simulink model "gm_parallel_8_prediction_and_cost_function"  (R2022a)
settings: Solver=FixedStepDiscrete  StartTime=0.0  StopTime=10.0  RelTol=1e-3
undefined symbols (not defined in the file or in its folder): f_c, L_d, L_q, L_x, L_y, p, psi_pm, R_ph
libraries: hdlmdlgenlib x42, hdlsllib x5
(part 3 of 7)

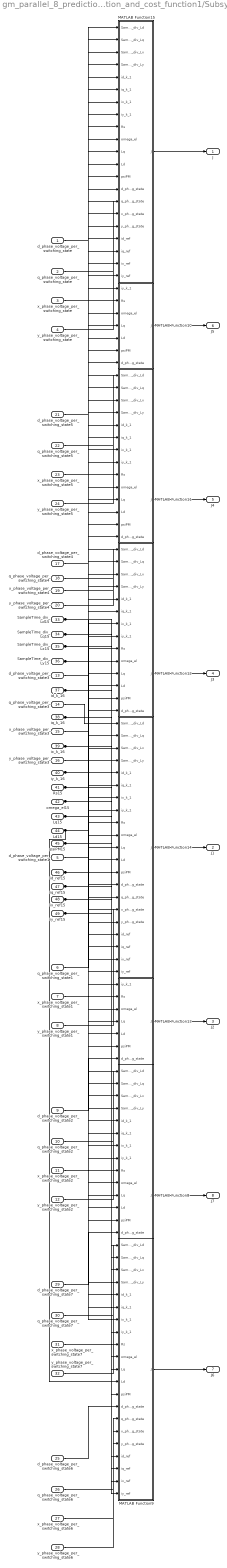
== system gm_parallel_8_prediction_and_cost_function/Prediction_and_cost_function1/Subsystem ==
  d_phase_voltage_per_switching_state : Inport  OutDataTypeStr=single  PortDimensions=1  SampleTime=1e-08
  q_phase_voltage_per_switching_state : Inport  Port=2  OutDataTypeStr=single  PortDimensions=1  SampleTime=1e-08
  x_phase_voltage_per_switching_state : Inport  Port=3  OutDataTypeStr=single  PortDimensions=1  SampleTime=1e-08
  y_phase_voltage_per_switching_state : Inport  Port=4  OutDataTypeStr=single  PortDimensions=1  SampleTime=1e-08
  d_phase_voltage_per_switching_state1 : Inport  Port=5  OutDataTypeStr=single  PortDimensions=1  SampleTime=1e-08
  q_phase_voltage_per_switching_state1 : Inport  Port=6  OutDataTypeStr=single  PortDimensions=1  SampleTime=1e-08
  x_phase_voltage_per_switching_state1 : Inport  Port=7  OutDataTypeStr=single  PortDimensions=1  SampleTime=1e-08
  y_phase_voltage_per_switching_state1 : Inport  Port=8  OutDataTypeStr=single  PortDimensions=1  SampleTime=1e-08
  d_phase_voltage_per_switching_state2 : Inport  Port=9  OutDataTypeStr=single  PortDimensions=1  SampleTime=1e-08
  q_phase_voltage_per_switching_state2 : Inport  Port=10  OutDataTypeStr=single  PortDimensions=1  SampleTime=1e-08
  x_phase_voltage_per_switching_state2 : Inport  Port=11  OutDataTypeStr=single  PortDimensions=1  SampleTime=1e-08
  y_phase_voltage_per_switching_state2 : Inport  Port=12  OutDataTypeStr=single  PortDimensions=1  SampleTime=1e-08
  d_phase_voltage_per_switching_state3 : Inport  Port=13  OutDataTypeStr=single  PortDimensions=1  SampleTime=1e-08
  q_phase_voltage_per_switching_state3 : Inport  Port=14  OutDataTypeStr=single  PortDimensions=1  SampleTime=1e-08
  x_phase_voltage_per_switching_state3 : Inport  Port=15  OutDataTypeStr=single  PortDimensions=1  SampleTime=1e-08
  y_phase_voltage_per_switching_state3 : Inport  Port=16  OutDataTypeStr=single  PortDimensions=1  SampleTime=1e-08
  d_phase_voltage_per_switching_state4 : Inport  Port=17  OutDataTypeStr=single  PortDimensions=1  SampleTime=1e-08
  q_phase_voltage_per_switching_state4 : Inport  Port=18  OutDataTypeStr=single  PortDimensions=1  SampleTime=1e-08
  x_phase_voltage_per_switching_state4 : Inport  Port=19  OutDataTypeStr=single  PortDimensions=1  SampleTime=1e-08
  y_phase_voltage_per_switching_state4 : Inport  Port=20  OutDataTypeStr=single  PortDimensions=1  SampleTime=1e-08
  d_phase_voltage_per_switching_state5 : Inport  Port=21  OutDataTypeStr=single  PortDimensions=1  SampleTime=1e-08
  q_phase_voltage_per_switching_state5 : Inport  Port=22  OutDataTypeStr=single  PortDimensions=1  SampleTime=1e-08
  x_phase_voltage_per_switching_state5 : Inport  Port=23  OutDataTypeStr=single  PortDimensions=1  SampleTime=1e-08
  y_phase_voltage_per_switching_state5 : Inport  Port=24  OutDataTypeStr=single  PortDimensions=1  SampleTime=1e-08
  d_phase_voltage_per_switching_state6 : Inport  Port=25  OutDataTypeStr=single  PortDimensions=1  SampleTime=1e-08
  q_phase_voltage_per_switching_state6 : Inport  Port=26  OutDataTypeStr=single  PortDimensions=1  SampleTime=1e-08
  x_phase_voltage_per_switching_state6 : Inport  Port=27  OutDataTypeStr=single  PortDimensions=1  SampleTime=1e-08
  y_phase_voltage_per_switching_state6 : Inport  Port=28  OutDataTypeStr=single  PortDimensions=1  SampleTime=1e-08
  d_phase_voltage_per_switching_state7 : Inport  Port=29  OutDataTypeStr=single  PortDimensions=1  SampleTime=1e-08
  q_phase_voltage_per_switching_state7 : Inport  Port=30  OutDataTypeStr=single  PortDimensions=1  SampleTime=1e-08
  x_phase_voltage_per_switching_state7 : Inport  Port=31  OutDataTypeStr=single  PortDimensions=1  SampleTime=1e-08
  y_phase_voltage_per_switching_state7 : Inport  Port=32  OutDataTypeStr=single  PortDimensions=1  SampleTime=1e-08
  SampleTime_div_Ld15 : Inport  Port=33  OutDataTypeStr=single  PortDimensions=1  SampleTime=1e-08
  SampleTime_div_Lq15 : Inport  Port=34  OutDataTypeStr=single  PortDimensions=1  SampleTime=1e-08
  SampleTime_div_Lx15 : Inport  Port=35  OutDataTypeStr=single  PortDimensions=1  SampleTime=1e-08
  SampleTime_div_Ly15 : Inport  Port=36  OutDataTypeStr=single  PortDimensions=1  SampleTime=1e-08
  id_k_16 : Inport  Port=37  OutDataTypeStr=single  PortDimensions=1  SampleTime=1e-08
  iq_k_16 : Inport  Port=38  OutDataTypeStr=single  PortDimensions=1  SampleTime=1e-08
  ix_k_16 : Inport  Port=39  OutDataTypeStr=single  PortDimensions=1  SampleTime=1e-08
  iy_k_16 : Inport  Port=40  OutDataTypeStr=single  PortDimensions=1  SampleTime=1e-08
  Rs15 : Inport  Port=41  OutDataTypeStr=single  PortDimensions=1  SampleTime=1e-08
  omega_el15 : Inport  Port=42  OutDataTypeStr=single  PortDimensions=1  SampleTime=1e-08
  Lq15 : Inport  Port=43  OutDataTypeStr=single  PortDimensions=1  SampleTime=1e-08
  Ld15 : Inport  Port=44  OutDataTypeStr=single  PortDimensions=1  SampleTime=1e-08
  psiPM15 : Inport  Port=45  OutDataTypeStr=single  PortDimensions=1  SampleTime=1e-08
  id_ref15 : Inport  Port=46  OutDataTypeStr=single  PortDimensions=1  SampleTime=1e-08
  iq_ref15 : Inport  Port=47  OutDataTypeStr=single  PortDimensions=1  SampleTime=1e-08
  ix_ref15 : Inport  Port=48  OutDataTypeStr=single  PortDimensions=1  SampleTime=1e-08
  iy_ref15 : Inport  Port=49  OutDataTypeStr=single  PortDimensions=1  SampleTime=1e-08
  MATLAB Function10 : Subsystem
  MATLAB Function11 : Subsystem
  MATLAB Function12 : Subsystem
  MATLAB Function13 : Subsystem
  MATLAB Function14 : Subsystem
  MATLAB Function15 : Subsystem
  MATLAB Function8 : Subsystem
  MATLAB Function9 : Subsystem
  J : Outport  SampleTime=1e-08
  J1 : Outport  Port=2  SampleTime=1e-08
  J2 : Outport  Port=3  SampleTime=1e-08
  J3 : Outport  Port=4  SampleTime=1e-08
  J4 : Outport  Port=5  SampleTime=1e-08
  J5 : Outport  Port=6  SampleTime=1e-08
  J6 : Outport  Port=7  SampleTime=1e-08
  J7 : Outport  Port=8  SampleTime=1e-08
  wires:
  MATLAB Function10/1(J) -> J5/1
  MATLAB Function11/1(J) -> J4/1
  MATLAB Function12/1(J) -> J3/1
  MATLAB Function13/1(J) -> J2/1
  MATLAB Function14/1(J) -> J1/1
  MATLAB Function15/1(J) -> J/1
  MATLAB Function8/1(J) -> J7/1
  MATLAB Function9/1(J) -> J6/1
  d_phase_voltage_per_switching_state/1 -> MATLAB Function15/14(d_phase_voltage_per_switching_state)
  q_phase_voltage_per_switching_state/1 -> MATLAB Function15/15(q_phase_voltage_per_switching_state)
  x_phase_voltage_per_switching_state/1 -> MATLAB Function15/16(x_phase_voltage_per_switching_state)
  y_phase_voltage_per_switching_state/1 -> MATLAB Function15/17(y_phase_voltage_per_switching_state)
  d_phase_voltage_per_switching_state1/1 -> MATLAB Function14/14(d_phase_voltage_per_switching_state)
  q_phase_voltage_per_switching_state1/1 -> MATLAB Function14/15(q_phase_voltage_per_switching_state)
  x_phase_voltage_per_switching_state1/1 -> MATLAB Function14/16(x_phase_voltage_per_switching_state)
  y_phase_voltage_per_switching_state1/1 -> MATLAB Function14/17(y_phase_voltage_per_switching_state)
  d_phase_voltage_per_switching_state2/1 -> MATLAB Function13/14(d_phase_voltage_per_switching_state)
  q_phase_voltage_per_switching_state2/1 -> MATLAB Function13/15(q_phase_voltage_per_switching_state)
  x_phase_voltage_per_switching_state2/1 -> MATLAB Function13/16(x_phase_voltage_per_switching_state)
  y_phase_voltage_per_switching_state2/1 -> MATLAB Function13/17(y_phase_voltage_per_switching_state)
  d_phase_voltage_per_switching_state3/1 -> MATLAB Function12/14(d_phase_voltage_per_switching_state)
  q_phase_voltage_per_switching_state3/1 -> MATLAB Function12/15(q_phase_voltage_per_switching_state)
  x_phase_voltage_per_switching_state3/1 -> MATLAB Function12/16(x_phase_voltage_per_switching_state)
  y_phase_voltage_per_switching_state3/1 -> MATLAB Function12/17(y_phase_voltage_per_switching_state)
  d_phase_voltage_per_switching_state4/1 -> MATLAB Function11/14(d_phase_voltage_per_switching_state)
  q_phase_voltage_per_switching_state4/1 -> MATLAB Function11/15(q_phase_voltage_per_switching_state)
  x_phase_voltage_per_switching_state4/1 -> MATLAB Function11/16(x_phase_voltage_per_switching_state)
  y_phase_voltage_per_switching_state4/1 -> MATLAB Function11/17(y_phase_voltage_per_switching_state)
  d_phase_voltage_per_switching_state5/1 -> MATLAB Function10/14(d_phase_voltage_per_switching_state)
  q_phase_voltage_per_switching_state5/1 -> MATLAB Function10/15(q_phase_voltage_per_switching_state)
  x_phase_voltage_per_switching_state5/1 -> MATLAB Function10/16(x_phase_voltage_per_switching_state)
  y_phase_voltage_per_switching_state5/1 -> MATLAB Function10/17(y_phase_voltage_per_switching_state)
  d_phase_voltage_per_switching_state6/1 -> MATLAB Function9/14(d_phase_voltage_per_switching_state)
  q_phase_voltage_per_switching_state6/1 -> MATLAB Function9/15(q_phase_voltage_per_switching_state)
  x_phase_voltage_per_switching_state6/1 -> MATLAB Function9/16(x_phase_voltage_per_switching_state)
  y_phase_voltage_per_switching_state6/1 -> MATLAB Function9/17(y_phase_voltage_per_switching_state)
  d_phase_voltage_per_switching_state7/1 -> MATLAB Function8/14(d_phase_voltage_per_switching_state)
  q_phase_voltage_per_switching_state7/1 -> MATLAB Function8/15(q_phase_voltage_per_switching_state)
  x_phase_voltage_per_switching_state7/1 -> MATLAB Function8/16(x_phase_voltage_per_switching_state)
  y_phase_voltage_per_switching_state7/1 -> MATLAB Function8/17(y_phase_voltage_per_switching_state)
  SampleTime_div_Ld15/1 -> MATLAB Function9/1(SampleTime_div_Ld), MATLAB Function8/1(SampleTime_div_Ld), MATLAB Function15/1(SampleTime_div_Ld), MATLAB Function14/1(SampleTime_div_Ld), MATLAB Function13/1(SampleTime_div_Ld), MATLAB Function12/1(SampleTime_div_Ld), MATLAB Function11/1(SampleTime_div_Ld), MATLAB Function10/1(SampleTime_div_Ld)
  SampleTime_div_Lq15/1 -> MATLAB Function9/2(SampleTime_div_Lq), MATLAB Function8/2(SampleTime_div_Lq), MATLAB Function15/2(SampleTime_div_Lq), MATLAB Function14/2(SampleTime_div_Lq), MATLAB Function13/2(SampleTime_div_Lq), MATLAB Function12/2(SampleTime_div_Lq), MATLAB Function11/2(SampleTime_div_Lq), MATLAB Function10/2(SampleTime_div_Lq)
  SampleTime_div_Lx15/1 -> MATLAB Function9/3(SampleTime_div_Lx), MATLAB Function8/3(SampleTime_div_Lx), MATLAB Function15/3(SampleTime_div_Lx), MATLAB Function14/3(SampleTime_div_Lx), MATLAB Function13/3(SampleTime_div_Lx), MATLAB Function12/3(SampleTime_div_Lx), MATLAB Function11/3(SampleTime_div_Lx), MATLAB Function10/3(SampleTime_div_Lx)
  SampleTime_div_Ly15/1 -> MATLAB Function9/4(SampleTime_div_Ly), MATLAB Function8/4(SampleTime_div_Ly), MATLAB Function15/4(SampleTime_div_Ly), MATLAB Function14/4(SampleTime_div_Ly), MATLAB Function13/4(SampleTime_div_Ly), MATLAB Function12/4(SampleTime_div_Ly), MATLAB Function11/4(SampleTime_div_Ly), MATLAB Function10/4(SampleTime_div_Ly)
  id_k_16/1 -> MATLAB Function9/5(id_k_1), MATLAB Function8/5(id_k_1), MATLAB Function15/5(id_k_1), MATLAB Function14/5(id_k_1), MATLAB Function13/5(id_k_1), MATLAB Function12/5(id_k_1), MATLAB Function11/5(id_k_1), MATLAB Function10/5(id_k_1)
  iq_k_16/1 -> MATLAB Function9/6(iq_k_1), MATLAB Function8/6(iq_k_1), MATLAB Function15/6(iq_k_1), MATLAB Function14/6(iq_k_1), MATLAB Function13/6(iq_k_1), MATLAB Function12/6(iq_k_1), MATLAB Function11/6(iq_k_1), MATLAB Function10/6(iq_k_1)
  ix_k_16/1 -> MATLAB Function9/7(ix_k_1), MATLAB Function8/7(ix_k_1), MATLAB Function15/7(ix_k_1), MATLAB Function14/7(ix_k_1), MATLAB Function13/7(ix_k_1), MATLAB Function12/7(ix_k_1), MATLAB Function11/7(ix_k_1), MATLAB Function10/7(ix_k_1)
  iy_k_16/1 -> MATLAB Function9/8(iy_k_1), MATLAB Function8/8(iy_k_1), MATLAB Function15/8(iy_k_1), MATLAB Function14/8(iy_k_1), MATLAB Function13/8(iy_k_1), MATLAB Function12/8(iy_k_1), MATLAB Function11/8(iy_k_1), MATLAB Function10/8(iy_k_1)
  Rs15/1 -> MATLAB Function9/9(Rs), MATLAB Function8/9(Rs), MATLAB Function15/9(Rs), MATLAB Function14/9(Rs), MATLAB Function13/9(Rs), MATLAB Function12/9(Rs), MATLAB Function11/9(Rs), MATLAB Function10/9(Rs)
  omega_el15/1 -> MATLAB Function9/10(omega_el), MATLAB Function8/10(omega_el), MATLAB Function15/10(omega_el), MATLAB Function14/10(omega_el), MATLAB Function13/10(omega_el), MATLAB Function12/10(omega_el), MATLAB Function11/10(omega_el), MATLAB Function10/10(omega_el)
  Lq15/1 -> MATLAB Function9/11(Lq), MATLAB Function8/11(Lq), MATLAB Function15/11(Lq), MATLAB Function14/11(Lq), MATLAB Function13/11(Lq), MATLAB Function12/11(Lq), MATLAB Function11/11(Lq), MATLAB Function10/11(Lq)
  Ld15/1 -> MATLAB Function9/12(Ld), MATLAB Function8/12(Ld), MATLAB Function15/12(Ld), MATLAB Function14/12(Ld), MATLAB Function13/12(Ld), MATLAB Function12/12(Ld), MATLAB Function11/12(Ld), MATLAB Function10/12(Ld)
  psiPM15/1 -> MATLAB Function9/13(psiPM), MATLAB Function8/13(psiPM), MATLAB Function15/13(psiPM), MATLAB Function14/13(psiPM), MATLAB Function13/13(psiPM), MATLAB Function12/13(psiPM), MATLAB Function11/13(psiPM), MATLAB Function10/13(psiPM)
  id_ref15/1 -> MATLAB Function9/18(id_ref), MATLAB Function8/18(id_ref), MATLAB Function15/18(id_ref), MATLAB Function14/18(id_ref), MATLAB Function13/18(id_ref), MATLAB Function12/18(id_ref), MATLAB Function11/18(id_ref), MATLAB Function10/18(id_ref)
  iq_ref15/1 -> MATLAB Function9/19(iq_ref), MATLAB Function8/19(iq_ref), MATLAB Function15/19(iq_ref), MATLAB Function14/19(iq_ref), MATLAB Function13/19(iq_ref), MATLAB Function12/19(iq_ref), MATLAB Function11/19(iq_ref), MATLAB Function10/19(iq_ref)
  ix_ref15/1 -> MATLAB Function9/20(ix_ref), MATLAB Function8/20(ix_ref), MATLAB Function15/20(ix_ref), MATLAB Function14/20(ix_ref), MATLAB Function13/20(ix_ref), MATLAB Function12/20(ix_ref), MATLAB Function11/20(ix_ref), MATLAB Function10/20(ix_ref)
  iy_ref15/1 -> MATLAB Function9/21(iy_ref), MATLAB Function8/21(iy_ref), MATLAB Function15/21(iy_ref), MATLAB Function14/21(iy_ref), MATLAB Function13/21(iy_ref), MATLAB Function12/21(iy_ref), MATLAB Function11/21(iy_ref), MATLAB Function10/21(iy_ref)

== system gm_parallel_8_prediction_and_cost_function/Prediction_and_cost_function2/Subsystem ==
  d_phase_voltage_per_switching_state : Inport
  q_phase_voltage_per_switching_state : Inport  Port=2
  x_phase_voltage_per_switching_state : Inport  Port=3
  y_phase_voltage_per_switching_state : Inport  Port=4
  d_phase_voltage_per_switching_state1 : Inport  Port=5
  q_phase_voltage_per_switching_state1 : Inport  Port=6
  x_phase_voltage_per_switching_state1 : Inport  Port=7
  y_phase_voltage_per_switching_state1 : Inport  Port=8
  d_phase_voltage_per_switching_state2 : Inport  Port=9
  q_phase_voltage_per_switching_state2 : Inport  Port=10
  x_phase_voltage_per_switching_state2 : Inport  Port=11
  y_phase_voltage_per_switching_state2 : Inport  Port=12
  d_phase_voltage_per_switching_state3 : Inport  Port=13
  q_phase_voltage_per_switching_state3 : Inport  Port=14
  x_phase_voltage_per_switching_state3 : Inport  Port=15
  y_phase_voltage_per_switching_state3 : Inport  Port=16
  d_phase_voltage_per_switching_state4 : Inport  Port=17
  q_phase_voltage_per_switching_state4 : Inport  Port=18
  x_phase_voltage_per_switching_state4 : Inport  Port=19
  y_phase_voltage_per_switching_state4 : Inport  Port=20
  d_phase_voltage_per_switching_state5 : Inport  Port=21
  q_phase_voltage_per_switching_state5 : Inport  Port=22
  x_phase_voltage_per_switching_state5 : Inport  Port=23
  y_phase_voltage_per_switching_state5 : Inport  Port=24
  d_phase_voltage_per_switching_state6 : Inport  Port=25
  q_phase_voltage_per_switching_state6 : Inport  Port=26
  x_phase_voltage_per_switching_state6 : Inport  Port=27
  y_phase_voltage_per_switching_state6 : Inport  Port=28
  d_phase_voltage_per_switching_state7 : Inport  Port=29
  q_phase_voltage_per_switching_state7 : Inport  Port=30
  x_phase_voltage_per_switching_state7 : Inport  Port=31
  y_phase_voltage_per_switching_state7 : Inport  Port=32
  SampleTime_div_Ld15 : Inport  Port=33
  SampleTime_div_Lq15 : Inport  Port=34
  SampleTime_div_Lx15 : Inport  Port=35
  SampleTime_div_Ly15 : Inport  Port=36
  id_k_16 : Inport  Port=37
  iq_k_16 : Inport  Port=38
  ix_k_16 : Inport  Port=39
  iy_k_16 : Inport  Port=40
  Rs15 : Inport  Port=41
  omega_el15 : Inport  Port=42
  Lq15 : Inport  Port=43
  Ld15 : Inport  Port=44
  psiPM15 : Inport  Port=45
  id_ref15 : Inport  Port=46
  iq_ref15 : Inport  Port=47
  ix_ref15 : Inport  Port=48
  iy_ref15 : Inport  Port=49
  MATLAB Function10 : MATLAB Function  TreatAsAtomicUnit=on  SystemSampleTime=1/100000000
  MATLAB Function11 : MATLAB Function  TreatAsAtomicUnit=on  SystemSampleTime=1/100000000
  MATLAB Function12 : MATLAB Function  TreatAsAtomicUnit=on  SystemSampleTime=1/100000000
  MATLAB Function13 : MATLAB Function  TreatAsAtomicUnit=on  SystemSampleTime=1/100000000
  MATLAB Function14 : MATLAB Function  TreatAsAtomicUnit=on  SystemSampleTime=1/100000000
  MATLAB Function15 : MATLAB Function  TreatAsAtomicUnit=on  SystemSampleTime=1/100000000
  MATLAB Function8 : MATLAB Function  TreatAsAtomicUnit=on  SystemSampleTime=1/100000000
  MATLAB Function9 : MATLAB Function  TreatAsAtomicUnit=on  SystemSampleTime=1/100000000
  J : Outport
  J1 : Outport  Port=2
  J2 : Outport  Port=3
  J3 : Outport  Port=4
  J4 : Outport  Port=5
  J5 : Outport  Port=6
  J6 : Outport  Port=7
  J7 : Outport  Port=8
  wires:
  id_k_16/1 -> MATLAB Function15/5(id_k_1), MATLAB Function14/5(id_k_1), MATLAB Function13/5(id_k_1), MATLAB Function12/5(id_k_1), MATLAB Function11/5(id_k_1), MATLAB Function10/5(id_k_1), MATLAB Function9/5(id_k_1), MATLAB Function8/5(id_k_1)
  iq_k_16/1 -> MATLAB Function15/6(iq_k_1), MATLAB Function14/6(iq_k_1), MATLAB Function13/6(iq_k_1), MATLAB Function12/6(iq_k_1), MATLAB Function11/6(iq_k_1), MATLAB Function10/6(iq_k_1), MATLAB Function9/6(iq_k_1), MATLAB Function8/6(iq_k_1)
  ix_k_16/1 -> MATLAB Function15/7(ix_k_1), MATLAB Function14/7(ix_k_1), MATLAB Function13/7(ix_k_1), MATLAB Function12/7(ix_k_1), MATLAB Function11/7(ix_k_1), MATLAB Function10/7(ix_k_1), MATLAB Function9/7(ix_k_1), MATLAB Function8/7(ix_k_1)
  iy_k_16/1 -> MATLAB Function15/8(iy_k_1), MATLAB Function14/8(iy_k_1), MATLAB Function13/8(iy_k_1), MATLAB Function12/8(iy_k_1), MATLAB Function11/8(iy_k_1), MATLAB Function10/8(iy_k_1), MATLAB Function9/8(iy_k_1), MATLAB Function8/8(iy_k_1)
  Ld15/1 -> MATLAB Function15/12(Ld), MATLAB Function14/12(Ld), MATLAB Function13/12(Ld), MATLAB Function12/12(Ld), MATLAB Function11/12(Ld), MATLAB Function10/12(Ld), MATLAB Function9/12(Ld), MATLAB Function8/12(Ld)
  id_ref15/1 -> MATLAB Function15/18(id_ref), MATLAB Function14/18(id_ref), MATLAB Function13/18(id_ref), MATLAB Function12/18(id_ref), MATLAB Function11/18(id_ref), MATLAB Function10/18(id_ref), MATLAB Function9/18(id_ref), MATLAB Function8/18(id_ref)
  iq_ref15/1 -> MATLAB Function15/19(iq_ref), MATLAB Function14/19(iq_ref), MATLAB Function13/19(iq_ref), MATLAB Function12/19(iq_ref), MATLAB Function11/19(iq_ref), MATLAB Function10/19(iq_ref), MATLAB Function9/19(iq_ref), MATLAB Function8/19(iq_ref)
  ix_ref15/1 -> MATLAB Function15/20(ix_ref), MATLAB Function14/20(ix_ref), MATLAB Function13/20(ix_ref), MATLAB Function12/20(ix_ref), MATLAB Function11/20(ix_ref), MATLAB Function10/20(ix_ref), MATLAB Function9/20(ix_ref), MATLAB Function8/20(ix_ref)
  q_phase_voltage_per_switching_state3/1 -> MATLAB Function12/15(q_phase_voltage_per_switching_state)
  y_phase_voltage_per_switching_state3/1 -> MATLAB Function12/17(y_phase_voltage_per_switching_state)
  q_phase_voltage_per_switching_state7/1 -> MATLAB Function8/15(q_phase_voltage_per_switching_state)
  MATLAB Function12/1(J) -> J3/1
  MATLAB Function9/1(J) -> J6/1
  x_phase_voltage_per_switching_state6/1 -> MATLAB Function9/16(x_phase_voltage_per_switching_state)
  y_phase_voltage_per_switching_state6/1 -> MATLAB Function9/17(y_phase_voltage_per_switching_state)
  q_phase_voltage_per_switching_state6/1 -> MATLAB Function9/15(q_phase_voltage_per_switching_state)
  y_phase_voltage_per_switching_state5/1 -> MATLAB Function10/17(y_phase_voltage_per_switching_state)
  MATLAB Function10/1(J) -> J5/1
  d_phase_voltage_per_switching_state5/1 -> MATLAB Function10/14(d_phase_voltage_per_switching_state)
  MATLAB Function15/1(J) -> J/1
  q_phase_voltage_per_switching_state/1 -> MATLAB Function15/15(q_phase_voltage_per_switching_state)
  x_phase_voltage_per_switching_state7/1 -> MATLAB Function8/16(x_phase_voltage_per_switching_state)
  SampleTime_div_Lq15/1 -> MATLAB Function15/2(SampleTime_div_Lq), MATLAB Function14/2(SampleTime_div_Lq), MATLAB Function13/2(SampleTime_div_Lq), MATLAB Function12/2(SampleTime_div_Lq), MATLAB Function11/2(SampleTime_div_Lq), MATLAB Function10/2(SampleTime_div_Lq), MATLAB Function9/2(SampleTime_div_Lq), MATLAB Function8/2(SampleTime_div_Lq)
  SampleTime_div_Ly15/1 -> MATLAB Function15/4(SampleTime_div_Ly), MATLAB Function14/4(SampleTime_div_Ly), MATLAB Function13/4(SampleTime_div_Ly), MATLAB Function12/4(SampleTime_div_Ly), MATLAB Function11/4(SampleTime_div_Ly), MATLAB Function10/4(SampleTime_div_Ly), MATLAB Function9/4(SampleTime_div_Ly), MATLAB Function8/4(SampleTime_div_Ly)
  SampleTime_div_Lx15/1 -> MATLAB Function15/3(SampleTime_div_Lx), MATLAB Function14/3(SampleTime_div_Lx), MATLAB Function13/3(SampleTime_div_Lx), MATLAB Function12/3(SampleTime_div_Lx), MATLAB Function11/3(SampleTime_div_Lx), MATLAB Function10/3(SampleTime_div_Lx), MATLAB Function9/3(SampleTime_div_Lx), MATLAB Function8/3(SampleTime_div_Lx)
  x_phase_voltage_per_switching_state5/1 -> MATLAB Function10/16(x_phase_voltage_per_switching_state)
  q_phase_voltage_per_switching_state4/1 -> MATLAB Function11/15(q_phase_voltage_per_switching_state)
  d_phase_voltage_per_switching_state4/1 -> MATLAB Function11/14(d_phase_voltage_per_switching_state)
  d_phase_voltage_per_switching_state7/1 -> MATLAB Function8/14(d_phase_voltage_per_switching_state)
  q_phase_voltage_per_switching_state5/1 -> MATLAB Function10/15(q_phase_voltage_per_switching_state)
  x_phase_voltage_per_switching_state/1 -> MATLAB Function15/16(x_phase_voltage_per_switching_state)
  y_phase_voltage_per_switching_state4/1 -> MATLAB Function11/17(y_phase_voltage_per_switching_state)
  MATLAB Function13/1(J) -> J2/1
  x_phase_voltage_per_switching_state2/1 -> MATLAB Function13/16(x_phase_voltage_per_switching_state)
  q_phase_voltage_per_switching_state2/1 -> MATLAB Function13/15(q_phase_voltage_per_switching_state)
  MATLAB Function8/1(J) -> J7/1
  MATLAB Function14/1(J) -> J1/1
  y_phase_voltage_per_switching_state1/1 -> MATLAB Function14/17(y_phase_voltage_per_switching_state)
  x_phase_voltage_per_switching_state4/1 -> MATLAB Function11/16(x_phase_voltage_per_switching_state)
  d_phase_voltage_per_switching_state2/1 -> MATLAB Function13/14(d_phase_voltage_per_switching_state)
  x_phase_voltage_per_switching_state3/1 -> MATLAB Function12/16(x_phase_voltage_per_switching_state)
  d_phase_voltage_per_switching_state/1 -> MATLAB Function15/14(d_phase_voltage_per_switching_state)
  d_phase_voltage_per_switching_state6/1 -> MATLAB Function9/14(d_phase_voltage_per_switching_state)
  d_phase_voltage_per_switching_state3/1 -> MATLAB Function12/14(d_phase_voltage_per_switching_state)
  psiPM15/1 -> MATLAB Function15/13(psiPM), MATLAB Function14/13(psiPM), MATLAB Function13/13(psiPM), MATLAB Function12/13(psiPM), MATLAB Function11/13(psiPM), MATLAB Function10/13(psiPM), MATLAB Function9/13(psiPM), MATLAB Function8/13(psiPM)
  omega_el15/1 -> MATLAB Function15/10(omega_el), MATLAB Function14/10(omega_el), MATLAB Function13/10(omega_el), MATLAB Function12/10(omega_el), MATLAB Function11/10(omega_el), MATLAB Function10/10(omega_el), MATLAB Function9/10(omega_el), MATLAB Function8/10(omega_el)
  iy_ref15/1 -> MATLAB Function15/21(iy_ref), MATLAB Function14/21(iy_ref), MATLAB Function13/21(iy_ref), MATLAB Function12/21(iy_ref), MATLAB Function11/21(iy_ref), MATLAB Function10/21(iy_ref), MATLAB Function9/21(iy_ref), MATLAB Function8/21(iy_ref)
  y_phase_voltage_per_switching_state7/1 -> MATLAB Function8/17(y_phase_voltage_per_switching_state)
  x_phase_voltage_per_switching_state1/1 -> MATLAB Function14/16(x_phase_voltage_per_switching_state)
  d_phase_voltage_per_switching_state1/1 -> MATLAB Function14/14(d_phase_voltage_per_switching_state)
  y_phase_voltage_per_switching_state2/1 -> MATLAB Function13/17(y_phase_voltage_per_switching_state)
  MATLAB Function11/1(J) -> J4/1
  Lq15/1 -> MATLAB Function15/11(Lq), MATLAB Function14/11(Lq), MATLAB Function13/11(Lq), MATLAB Function12/11(Lq), MATLAB Function11/11(Lq), MATLAB Function10/11(Lq), MATLAB Function9/11(Lq), MATLAB Function8/11(Lq)
  y_phase_voltage_per_switching_state/1 -> MATLAB Function15/17(y_phase_voltage_per_switching_state)
  Rs15/1 -> MATLAB Function15/9(Rs), MATLAB Function14/9(Rs), MATLAB Function13/9(Rs), MATLAB Function12/9(Rs), MATLAB Function11/9(Rs), MATLAB Function10/9(Rs), MATLAB Function9/9(Rs), MATLAB Function8/9(Rs)
  SampleTime_div_Ld15/1 -> MATLAB Function15/1(SampleTime_div_Ld), MATLAB Function14/1(SampleTime_div_Ld), MATLAB Function13/1(SampleTime_div_Ld), MATLAB Function12/1(SampleTime_div_Ld), MATLAB Function11/1(SampleTime_div_Ld), MATLAB Function10/1(SampleTime_div_Ld), MATLAB Function9/1(SampleTime_div_Ld), MATLAB Function8/1(SampleTime_div_Ld)
  q_phase_voltage_per_switching_state1/1 -> MATLAB Function14/15(q_phase_voltage_per_switching_state)

== system gm_parallel_8_prediction_and_cost_function/Prediction_and_cost_function1/Detect Rise Positive/Positive ==
  u : Inport  OutDataTypeStr=boolean  SampleTime=1e-08
  Compare : RelationalOperator  Operator=>  OutDataTypeStr=boolean  ZeroCross=off
  Constant : Constant  DisableCoverage=on  Value=0  OutDataTypeStr=Inherit: Inherit via back propagation  SampleTime=-1  PreserveConstantTs=on
  y : Outport  SampleTime=1e-08
  wires:
  Compare/1 -> y/1
  Constant/1 -> Compare/2
  u/1 -> Compare/1

== system gm_parallel_8_prediction_and_cost_function/Prediction_and_cost_function1/Detect Rise Positive1/Positive ==
  u : Inport  OutDataTypeStr=boolean  SampleTime=1e-08
  Compare : RelationalOperator  Operator=>  OutDataTypeStr=boolean  ZeroCross=off
  Constant : Constant  DisableCoverage=on  Value=0  OutDataTypeStr=Inherit: Inherit via back propagation  SampleTime=-1  PreserveConstantTs=on
  y : Outport  SampleTime=1e-08
  wires:
  Compare/1 -> y/1
  Constant/1 -> Compare/2
  u/1 -> Compare/1

== system gm_parallel_8_prediction_and_cost_function/Prediction_and_cost_function1/Detect Rise Positive2/Positive ==
  u : Inport  OutDataTypeStr=boolean  SampleTime=1e-08
  Compare : RelationalOperator  Operator=>  OutDataTypeStr=boolean  ZeroCross=off
  Constant : Constant  DisableCoverage=on  Value=0  OutDataTypeStr=Inherit: Inherit via back propagation  SampleTime=-1  PreserveConstantTs=on
  y : Outport  SampleTime=1e-08
  wires:
  Compare/1 -> y/1
  Constant/1 -> Compare/2
  u/1 -> Compare/1

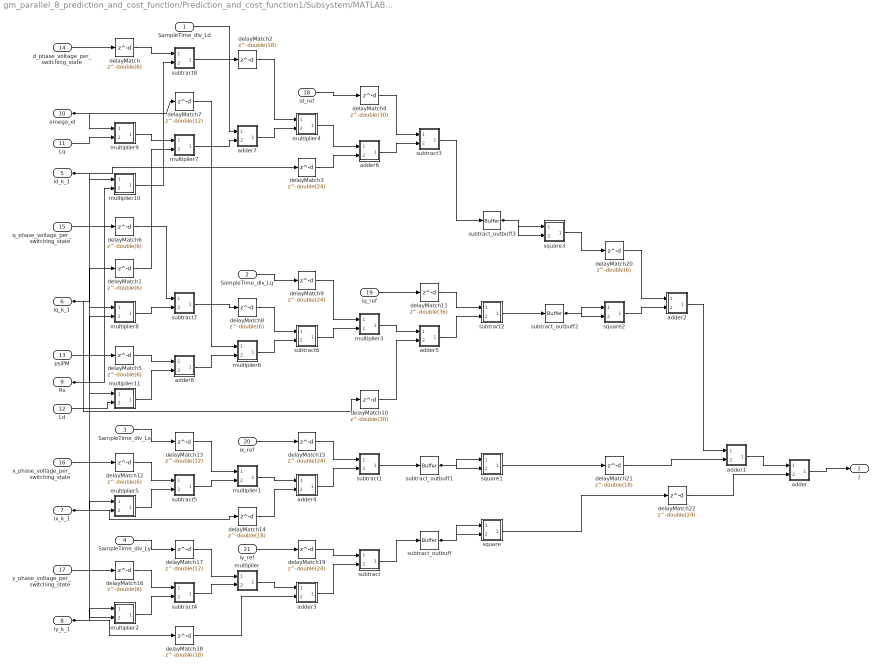
== system gm_parallel_8_prediction_and_cost_function/Prediction_and_cost_function1/Subsystem/MATLAB Function10 ==
  SampleTime_div_Ld : Inport  OutDataTypeStr=single  PortDimensions=1  SampleTime=1e-08
  SampleTime_div_Lq : Inport  Port=2  OutDataTypeStr=single  PortDimensions=1  SampleTime=1e-08
  SampleTime_div_Lx : Inport  Port=3  OutDataTypeStr=single  PortDimensions=1  SampleTime=1e-08
  SampleTime_div_Ly : Inport  Port=4  OutDataTypeStr=single  PortDimensions=1  SampleTime=1e-08
  id_k_1 : Inport  Port=5  OutDataTypeStr=single  PortDimensions=1  SampleTime=1e-08
  iq_k_1 : Inport  Port=6  OutDataTypeStr=single  PortDimensions=1  SampleTime=1e-08
  ix_k_1 : Inport  Port=7  OutDataTypeStr=single  PortDimensions=1  SampleTime=1e-08
  iy_k_1 : Inport  Port=8  OutDataTypeStr=single  PortDimensions=1  SampleTime=1e-08
  Rs : Inport  Port=9  OutDataTypeStr=single  PortDimensions=1  SampleTime=1e-08
  omega_el : Inport  Port=10  OutDataTypeStr=single  PortDimensions=1  SampleTime=1e-08
  Lq : Inport  Port=11  OutDataTypeStr=single  PortDimensions=1  SampleTime=1e-08
  Ld : Inport  Port=12  OutDataTypeStr=single  PortDimensions=1  SampleTime=1e-08
  psiPM : Inport  Port=13  OutDataTypeStr=single  PortDimensions=1  SampleTime=1e-08
  d_phase_voltage_per_switching_state : Inport  Port=14  OutDataTypeStr=single  PortDimensions=1  SampleTime=1e-08
  q_phase_voltage_per_switching_state : Inport  Port=15  OutDataTypeStr=single  PortDimensions=1  SampleTime=1e-08
  x_phase_voltage_per_switching_state : Inport  Port=16  OutDataTypeStr=single  PortDimensions=1  SampleTime=1e-08
  y_phase_voltage_per_switching_state : Inport  Port=17  OutDataTypeStr=single  PortDimensions=1  SampleTime=1e-08
  id_ref : Inport  Port=18  OutDataTypeStr=single  PortDimensions=1  SampleTime=1e-08
  iq_ref : Inport  Port=19  OutDataTypeStr=single  PortDimensions=1  SampleTime=1e-08
  ix_ref : Inport  Port=20  OutDataTypeStr=single  PortDimensions=1  SampleTime=1e-08
  iy_ref : Inport  Port=21  OutDataTypeStr=single  PortDimensions=1  SampleTime=1e-08
  adder : Subsystem
      mask Display: disp('NFP\nadd');
  adder1 : Subsystem
      mask Display: disp('NFP\nadd');
  adder2 : Subsystem
      mask Display: disp('NFP\nadd');
  adder3 : Subsystem
      mask Display: disp('NFP\nadd');
  adder4 : Subsystem
      mask Display: disp('NFP\nadd');
  adder5 : Subsystem
      mask Display: disp('NFP\nadd');
  adder6 : Subsystem
      mask Display: disp('NFP\nadd');
  adder7 : Subsystem
      mask Display: disp('NFP\nadd');
  adder8 : Subsystem
      mask Display: disp('NFP\nadd');
  delayMatch{,1,5..6,8,12,16,20} (8 alike) : Delay  DelayLength=double(6)  InitialCondition=0  SampleTime=1e-08
  delayMatch10 : Delay  DelayLength=double(30)  InitialCondition=0  SampleTime=1e-08
  delayMatch11 : Delay  DelayLength=double(36)  InitialCondition=0  SampleTime=1e-08
  delayMatch13 : Delay  DelayLength=double(12)  InitialCondition=0  SampleTime=1e-08
  delayMatch{2,14,18,21} (4 alike) : Delay  DelayLength=double(18)  InitialCondition=0  SampleTime=1e-08
  delayMatch{3,9,15,19,22} (5 alike) : Delay  DelayLength=double(24)  InitialCondition=0  SampleTime=1e-08
  delayMatch17 : Delay  DelayLength=double(12)  InitialCondition=0  SampleTime=1e-08
  delayMatch4 : Delay  DelayLength=double(30)  InitialCondition=0  SampleTime=1e-08
  delayMatch7 : Delay  DelayLength=double(12)  InitialCondition=0  SampleTime=1e-08
  multiplier : Subsystem
      mask Display: disp('NFP\nmul');
  multiplier1 : Subsystem
      mask Display: disp('NFP\nmul');
  multiplier10 : Subsystem
      mask Display: disp('NFP\nmul');
  multiplier11 : Subsystem
      mask Display: disp('NFP\nmul');
  multiplier2 : Subsystem
      mask Display: disp('NFP\nmul');
  multiplier3 : Subsystem
      mask Display: disp('NFP\nmul');
  multiplier4 : Subsystem
      mask Display: disp('NFP\nmul');
  multiplier5 : Subsystem
      mask Display: disp('NFP\nmul');
  multiplier6 : Subsystem
      mask Display: disp('NFP\nmul');
  multiplier7 : Subsystem
      mask Display: disp('NFP\nmul');
  multiplier8 : Subsystem
      mask Display: disp('NFP\nmul');
  multiplier9 : Subsystem
      mask Display: disp('NFP\nmul');
  square : Subsystem
      mask Display: disp('NFP\nmul');
  square1 : Subsystem
      mask Display: disp('NFP\nmul');
  square2 : Subsystem
      mask Display: disp('NFP\nmul');
  square3 : Subsystem
      mask Display: disp('NFP\nmul');
  subtract : Subsystem
      mask Display: disp('NFP\nadd');
  subtract1 : Subsystem
      mask Display: disp('NFP\nadd');
  subtract2 : Subsystem
      mask Display: disp('NFP\nadd');
  subtract3 : Subsystem
      mask Display: disp('NFP\nadd');
  subtract4 : Subsystem
      mask Display: disp('NFP\nadd');
  subtract5 : Subsystem
      mask Display: disp('NFP\nadd');
  subtract6 : Subsystem
      mask Display: disp('NFP\nadd');
  subtract7 : Subsystem
      mask Display: disp('NFP\nadd');
  subtract8 : Subsystem
      mask Display: disp('NFP\nadd');
  subtract_outbuff{,1..3} (4 alike) : hdlmdlgenlib/Buffer
      settings: SourceProductBaseCode=SL
  J : Outport  SampleTime=1e-08  VectorParamsAs1DForOutWhenUnconnected=off
  wires:
  delayMatch2/1 -> multiplier4/1(In1)
  delayMatch9/1 -> multiplier3/1(In1)
  delayMatch13/1 -> multiplier1/1(In1)
  delayMatch17/1 -> multiplier/1(In1)
  delayMatch3/1 -> adder6/2(In2)
  delayMatch1/1 -> multiplier7/2(In2)
  delayMatch14/1 -> adder4/2(In2)
  delayMatch18/1 -> adder3/2(In2)
  delayMatch7/1 -> multiplier6/1(In1)
  delayMatch5/1 -> adder8/1(In1)
  delayMatch/1 -> subtract8/1(In1)
  delayMatch6/1 -> subtract7/1(In1)
  delayMatch12/1 -> subtract5/1(In1)
  delayMatch16/1 -> subtract4/1(In1)
  delayMatch4/1 -> subtract3/1(In1)
  delayMatch11/1 -> subtract2/1(In1)
  delayMatch15/1 -> subtract1/1(In1)
  delayMatch19/1 -> subtract/1(In1)
  delayMatch22/1 -> adder/2(In2)
  subtract_outbuff/1 -> square/2(In2), square/1(In1)
  delayMatch21/1 -> adder1/2(In2)
  subtract_outbuff1/1 -> square1/2(In2), square1/1(In1)
  delayMatch20/1 -> adder2/1(In1)
  subtract_outbuff2/1 -> square2/2(In2), square2/1(In1)
  subtract_outbuff3/1 -> square3/2(In2), square3/1(In1)
  delayMatch8/1 -> subtract6/1(In1)
  adder/1(Out1) -> J/1
  square/1(Out1) -> delayMatch22/1
  adder1/1(Out1) -> adder/1(In1)
  subtract/1(Out1) -> subtract_outbuff/1
  square1/1(Out1) -> delayMatch21/1
  adder2/1(Out1) -> adder1/1(In1)
  adder3/1(Out1) -> subtract/2(In2)
  subtract1/1(Out1) -> subtract_outbuff1/1
  square2/1(Out1) -> adder2/2(In2)
  square3/1(Out1) -> delayMatch20/1
  multiplier/1(Out1) -> adder3/1(In1)
  adder4/1(Out1) -> subtract1/2(In2)
  subtract2/1(Out1) -> subtract_outbuff2/1
  subtract3/1(Out1) -> subtract_outbuff3/1
  subtract4/1(Out1) -> multiplier/2(In2)
  multiplier1/1(Out1) -> adder4/1(In1)
  adder5/1(Out1) -> subtract2/2(In2)
  adder6/1(Out1) -> subtract3/2(In2)
  multiplier2/1(Out1) -> subtract4/2(In2)
  subtract5/1(Out1) -> multiplier1/2(In2)
  multiplier3/1(Out1) -> adder5/1(In1)
  multiplier4/1(Out1) -> adder6/1(In1)
  multiplier5/1(Out1) -> subtract5/2(In2)
  subtract6/1(Out1) -> multiplier3/2(In2)
  adder7/1(Out1) -> multiplier4/2(In2)
  multiplier6/1(Out1) -> subtract6/2(In2)
  subtract7/1(Out1) -> delayMatch8/1
  multiplier7/1(Out1) -> adder7/2(In2)
  subtract8/1(Out1) -> adder7/1(In1)
  adder8/1(Out1) -> multiplier6/2(In2)
  multiplier8/1(Out1) -> subtract7/2(In2)
  multiplier9/1(Out1) -> multiplier7/1(In1)
  multiplier10/1(Out1) -> subtract8/2(In2)
  multiplier11/1(Out1) -> adder8/2(In2)
  delayMatch10/1 -> adder5/2(In2)
  SampleTime_div_Ld/1 -> delayMatch2/1
  SampleTime_div_Lq/1 -> delayMatch9/1
  SampleTime_div_Lx/1 -> delayMatch13/1
  SampleTime_div_Ly/1 -> delayMatch17/1
  id_k_1/1 -> delayMatch3/1, multiplier11/1(In1), multiplier10/1(In1)
  iq_k_1/1 -> delayMatch10/1, delayMatch1/1, multiplier8/1(In1)
  ix_k_1/1 -> delayMatch14/1, multiplier5/1(In1)
  iy_k_1/1 -> delayMatch18/1, multiplier2/1(In1)
  Rs/1 -> multiplier10/2(In2), multiplier8/2(In2), multiplier5/2(In2), multiplier2/2(In2)
  omega_el/1 -> delayMatch7/1, multiplier9/1(In1)
  Lq/1 -> multiplier9/2(In2)
  Ld/1 -> multiplier11/2(In2)
  psiPM/1 -> delayMatch5/1
  d_phase_voltage_per_switching_state/1 -> delayMatch/1
  q_phase_voltage_per_switching_state/1 -> delayMatch6/1
  x_phase_voltage_per_switching_state/1 -> delayMatch12/1
  y_phase_voltage_per_switching_state/1 -> delayMatch16/1
  id_ref/1 -> delayMatch4/1
  iq_ref/1 -> delayMatch11/1
  ix_ref/1 -> delayMatch15/1
  iy_ref/1 -> delayMatch19/1

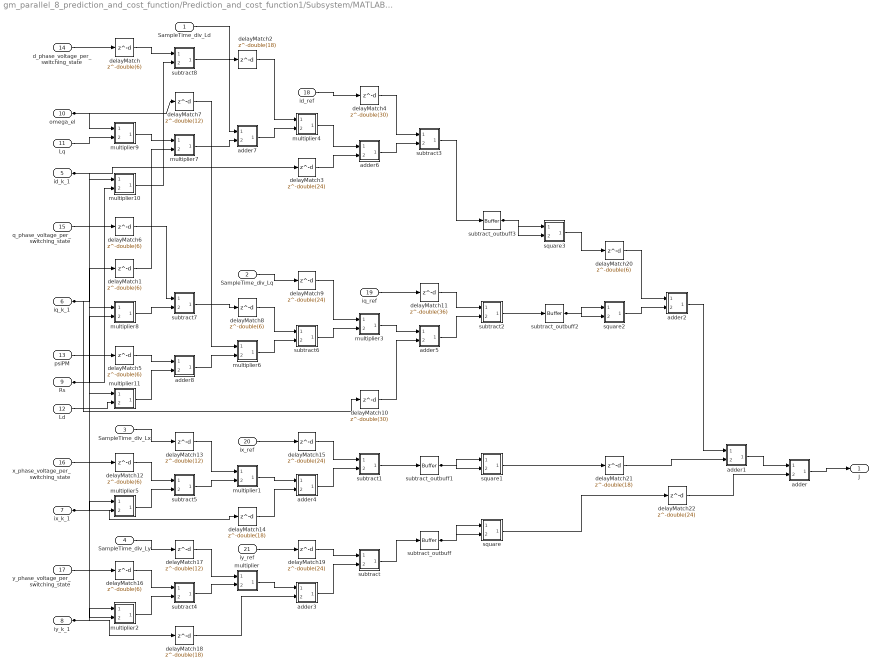
== system gm_parallel_8_prediction_and_cost_function/Prediction_and_cost_function1/Subsystem/MATLAB Function11 ==
  SampleTime_div_Ld : Inport  OutDataTypeStr=single  PortDimensions=1  SampleTime=1e-08
  SampleTime_div_Lq : Inport  Port=2  OutDataTypeStr=single  PortDimensions=1  SampleTime=1e-08
  SampleTime_div_Lx : Inport  Port=3  OutDataTypeStr=single  PortDimensions=1  SampleTime=1e-08
  SampleTime_div_Ly : Inport  Port=4  OutDataTypeStr=single  PortDimensions=1  SampleTime=1e-08
  id_k_1 : Inport  Port=5  OutDataTypeStr=single  PortDimensions=1  SampleTime=1e-08
  iq_k_1 : Inport  Port=6  OutDataTypeStr=single  PortDimensions=1  SampleTime=1e-08
  ix_k_1 : Inport  Port=7  OutDataTypeStr=single  PortDimensions=1  SampleTime=1e-08
  iy_k_1 : Inport  Port=8  OutDataTypeStr=single  PortDimensions=1  SampleTime=1e-08
  Rs : Inport  Port=9  OutDataTypeStr=single  PortDimensions=1  SampleTime=1e-08
  omega_el : Inport  Port=10  OutDataTypeStr=single  PortDimensions=1  SampleTime=1e-08
  Lq : Inport  Port=11  OutDataTypeStr=single  PortDimensions=1  SampleTime=1e-08
  Ld : Inport  Port=12  OutDataTypeStr=single  PortDimensions=1  SampleTime=1e-08
  psiPM : Inport  Port=13  OutDataTypeStr=single  PortDimensions=1  SampleTime=1e-08
  d_phase_voltage_per_switching_state : Inport  Port=14  OutDataTypeStr=single  PortDimensions=1  SampleTime=1e-08
  q_phase_voltage_per_switching_state : Inport  Port=15  OutDataTypeStr=single  PortDimensions=1  SampleTime=1e-08
  x_phase_voltage_per_switching_state : Inport  Port=16  OutDataTypeStr=single  PortDimensions=1  SampleTime=1e-08
  y_phase_voltage_per_switching_state : Inport  Port=17  OutDataTypeStr=single  PortDimensions=1  SampleTime=1e-08
  id_ref : Inport  Port=18  OutDataTypeStr=single  PortDimensions=1  SampleTime=1e-08
  iq_ref : Inport  Port=19  OutDataTypeStr=single  PortDimensions=1  SampleTime=1e-08
  ix_ref : Inport  Port=20  OutDataTypeStr=single  PortDimensions=1  SampleTime=1e-08
  iy_ref : Inport  Port=21  OutDataTypeStr=single  PortDimensions=1  SampleTime=1e-08
  adder : Subsystem
      mask Display: disp('NFP\nadd');
  adder1 : Subsystem
      mask Display: disp('NFP\nadd');
  adder2 : Subsystem
      mask Display: disp('NFP\nadd');
  adder3 : Subsystem
      mask Display: disp('NFP\nadd');
  adder4 : Subsystem
      mask Display: disp('NFP\nadd');
  adder5 : Subsystem
      mask Display: disp('NFP\nadd');
  adder6 : Subsystem
      mask Display: disp('NFP\nadd');
  adder7 : Subsystem
      mask Display: disp('NFP\nadd');
  adder8 : Subsystem
      mask Display: disp('NFP\nadd');
  delayMatch{,1,5..6,8,12,16,20} (8 alike) : Delay  DelayLength=double(6)  InitialCondition=0  SampleTime=1e-08
  delayMatch10 : Delay  DelayLength=double(30)  InitialCondition=0  SampleTime=1e-08
  delayMatch11 : Delay  DelayLength=double(36)  InitialCondition=0  SampleTime=1e-08
  delayMatch13 : Delay  DelayLength=double(12)  InitialCondition=0  SampleTime=1e-08
  delayMatch{2,14,18,21} (4 alike) : Delay  DelayLength=double(18)  InitialCondition=0  SampleTime=1e-08
  delayMatch{3,9,15,19,22} (5 alike) : Delay  DelayLength=double(24)  InitialCondition=0  SampleTime=1e-08
  delayMatch17 : Delay  DelayLength=double(12)  InitialCondition=0  SampleTime=1e-08
  delayMatch4 : Delay  DelayLength=double(30)  InitialCondition=0  SampleTime=1e-08
  delayMatch7 : Delay  DelayLength=double(12)  InitialCondition=0  SampleTime=1e-08
  multiplier : Subsystem
      mask Display: disp('NFP\nmul');
  multiplier1 : Subsystem
      mask Display: disp('NFP\nmul');
  multiplier10 : Subsystem
      mask Display: disp('NFP\nmul');
  multiplier11 : Subsystem
      mask Display: disp('NFP\nmul');
  multiplier2 : Subsystem
      mask Display: disp('NFP\nmul');
  multiplier3 : Subsystem
      mask Display: disp('NFP\nmul');
  multiplier4 : Subsystem
      mask Display: disp('NFP\nmul');
  multiplier5 : Subsystem
      mask Display: disp('NFP\nmul');
  multiplier6 : Subsystem
      mask Display: disp('NFP\nmul');
  multiplier7 : Subsystem
      mask Display: disp('NFP\nmul');
  multiplier8 : Subsystem
      mask Display: disp('NFP\nmul');
  multiplier9 : Subsystem
      mask Display: disp('NFP\nmul');
  square : Subsystem
      mask Display: disp('NFP\nmul');
  square1 : Subsystem
      mask Display: disp('NFP\nmul');
  square2 : Subsystem
      mask Display: disp('NFP\nmul');
  square3 : Subsystem
      mask Display: disp('NFP\nmul');
  subtract : Subsystem
      mask Display: disp('NFP\nadd');
  subtract1 : Subsystem
      mask Display: disp('NFP\nadd');
  subtract2 : Subsystem
      mask Display: disp('NFP\nadd');
  subtract3 : Subsystem
      mask Display: disp('NFP\nadd');
  subtract4 : Subsystem
      mask Display: disp('NFP\nadd');
  subtract5 : Subsystem
      mask Display: disp('NFP\nadd');
  subtract6 : Subsystem
      mask Display: disp('NFP\nadd');
  subtract7 : Subsystem
      mask Display: disp('NFP\nadd');
  subtract8 : Subsystem
      mask Display: disp('NFP\nadd');
  subtract_outbuff{,1..3} (4 alike) : hdlmdlgenlib/Buffer
      settings: SourceProductBaseCode=SL
  J : Outport  SampleTime=1e-08  VectorParamsAs1DForOutWhenUnconnected=off
  wires:
  iy_ref/1 -> delayMatch19/1
  ix_ref/1 -> delayMatch15/1
  iq_ref/1 -> delayMatch11/1
  id_ref/1 -> delayMatch4/1
  y_phase_voltage_per_switching_state/1 -> delayMatch16/1
  x_phase_voltage_per_switching_state/1 -> delayMatch12/1
  q_phase_voltage_per_switching_state/1 -> delayMatch6/1
  d_phase_voltage_per_switching_state/1 -> delayMatch/1
  psiPM/1 -> delayMatch5/1
  Ld/1 -> multiplier11/2(In2)
  Lq/1 -> multiplier9/2(In2)
  omega_el/1 -> multiplier9/1(In1), delayMatch7/1
  Rs/1 -> multiplier2/2(In2), multiplier5/2(In2), multiplier8/2(In2), multiplier10/2(In2)
  iy_k_1/1 -> multiplier2/1(In1), delayMatch18/1
  ix_k_1/1 -> multiplier5/1(In1), delayMatch14/1
  iq_k_1/1 -> multiplier8/1(In1), delayMatch1/1, delayMatch10/1
  id_k_1/1 -> multiplier10/1(In1), multiplier11/1(In1), delayMatch3/1
  SampleTime_div_Ly/1 -> delayMatch17/1
  SampleTime_div_Lx/1 -> delayMatch13/1
  SampleTime_div_Lq/1 -> delayMatch9/1
  SampleTime_div_Ld/1 -> delayMatch2/1
  delayMatch10/1 -> adder5/2(In2)
  multiplier11/1(Out1) -> adder8/2(In2)
  multiplier10/1(Out1) -> subtract8/2(In2)
  multiplier9/1(Out1) -> multiplier7/1(In1)
  multiplier8/1(Out1) -> subtract7/2(In2)
  adder8/1(Out1) -> multiplier6/2(In2)
  subtract8/1(Out1) -> adder7/1(In1)
  multiplier7/1(Out1) -> adder7/2(In2)
  subtract7/1(Out1) -> delayMatch8/1
  multiplier6/1(Out1) -> subtract6/2(In2)
  adder7/1(Out1) -> multiplier4/2(In2)
  subtract6/1(Out1) -> multiplier3/2(In2)
  multiplier5/1(Out1) -> subtract5/2(In2)
  multiplier4/1(Out1) -> adder6/1(In1)
  multiplier3/1(Out1) -> adder5/1(In1)
  subtract5/1(Out1) -> multiplier1/2(In2)
  multiplier2/1(Out1) -> subtract4/2(In2)
  adder6/1(Out1) -> subtract3/2(In2)
  adder5/1(Out1) -> subtract2/2(In2)
  multiplier1/1(Out1) -> adder4/1(In1)
  subtract4/1(Out1) -> multiplier/2(In2)
  subtract3/1(Out1) -> subtract_outbuff3/1
  subtract2/1(Out1) -> subtract_outbuff2/1
  adder4/1(Out1) -> subtract1/2(In2)
  multiplier/1(Out1) -> adder3/1(In1)
  square3/1(Out1) -> delayMatch20/1
  square2/1(Out1) -> adder2/2(In2)
  subtract1/1(Out1) -> subtract_outbuff1/1
  adder3/1(Out1) -> subtract/2(In2)
  adder2/1(Out1) -> adder1/1(In1)
  square1/1(Out1) -> delayMatch21/1
  subtract/1(Out1) -> subtract_outbuff/1
  adder1/1(Out1) -> adder/1(In1)
  square/1(Out1) -> delayMatch22/1
  adder/1(Out1) -> J/1
  delayMatch8/1 -> subtract6/1(In1)
  subtract_outbuff3/1 -> square3/1(In1), square3/2(In2)
  subtract_outbuff2/1 -> square2/1(In1), square2/2(In2)
  delayMatch20/1 -> adder2/1(In1)
  subtract_outbuff1/1 -> square1/1(In1), square1/2(In2)
  delayMatch21/1 -> adder1/2(In2)
  subtract_outbuff/1 -> square/1(In1), square/2(In2)
  delayMatch22/1 -> adder/2(In2)
  delayMatch19/1 -> subtract/1(In1)
  delayMatch15/1 -> subtract1/1(In1)
  delayMatch11/1 -> subtract2/1(In1)
  delayMatch4/1 -> subtract3/1(In1)
  delayMatch16/1 -> subtract4/1(In1)
  delayMatch12/1 -> subtract5/1(In1)
  delayMatch6/1 -> subtract7/1(In1)
  delayMatch/1 -> subtract8/1(In1)
  delayMatch5/1 -> adder8/1(In1)
  delayMatch7/1 -> multiplier6/1(In1)
  delayMatch18/1 -> adder3/2(In2)
  delayMatch14/1 -> adder4/2(In2)
  delayMatch1/1 -> multiplier7/2(In2)
  delayMatch3/1 -> adder6/2(In2)
  delayMatch17/1 -> multiplier/1(In1)
  delayMatch13/1 -> multiplier1/1(In1)
  delayMatch9/1 -> multiplier3/1(In1)
  delayMatch2/1 -> multiplier4/1(In1)
